simulink model "Switchvideo_orientation"  (R2024a)
settings: Solver=FixedStepAuto  StartTime=0.0  StopTime=inf  RelTol=1e-3
undefined symbols (not defined in the file): VideoDirection
settings Model: Creator=Sasha  LastModifiedBy=quentinlandon

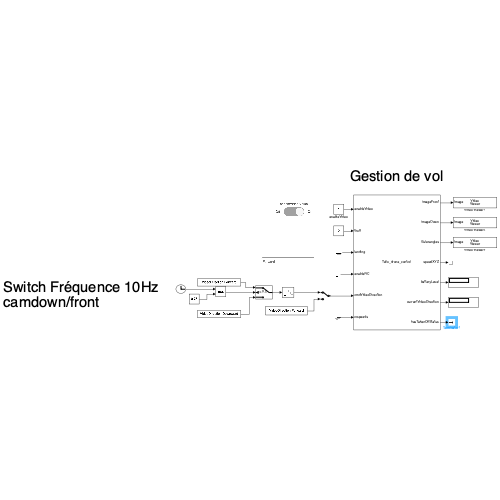
[thumbnail: Simulink's stored preview of the top-level diagram]
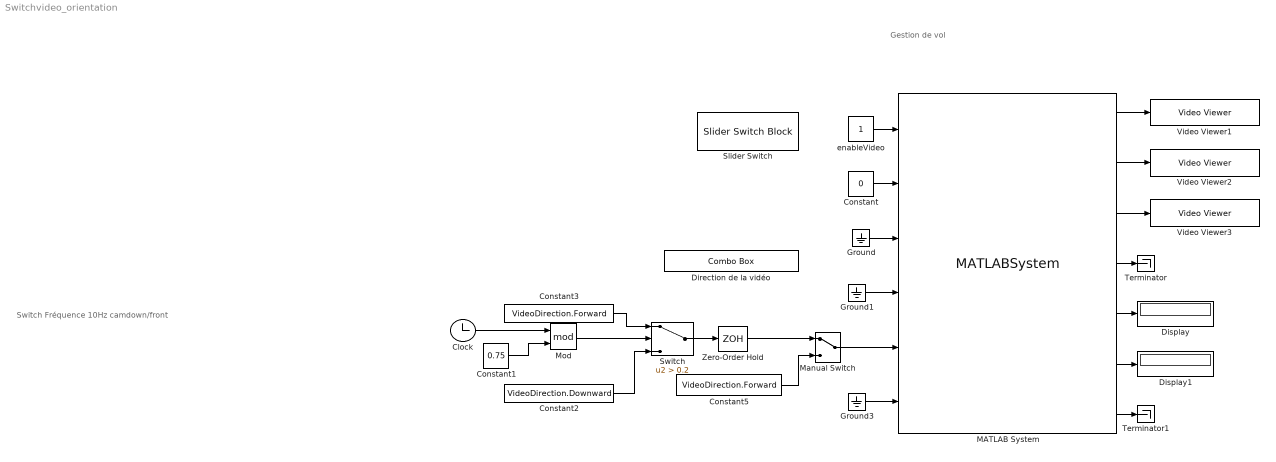
== system Switchvideo_orientation ==
  note: Gestion de vol
  note: Switch Fréquence 10Hz camdown/front
  Clock : Clock
  Constant : Constant  Value=0
  Constant1 : Constant  Value=0.75
  Constant2 : Constant  Value=VideoDirection.Downward
  Constant3 : Constant  Value=VideoDirection.Forward
  Constant5 : Constant  Value=VideoDirection.Forward
  Direction de la vidéo : ComboBox  LabelPosition=Hide  SelectedLabel=Forward  UseEnumeratedDataType=on  EnumeratedDataType=VideoDirection
      settings: Values={{'Forward', 'Downward', 'Both'}, [0 1 2]}
  Display : Display
  Display1 : Display
  Ground : Ground
  Ground1 : Ground
  Ground3 : Ground
  MATLAB System : MATLABSystem  System=Tello_drone_control  droneIP=127.0.0.1  SimulateUsing=Interpreted execution
      mask Type: Tello_drone_control
      mask Display:
      | disp('Tello_drone_control');
      | port_label('input',1,'enableVideo');
      | port_label('input',2,'tkoff');
      | port_label('input',3,'landing');
      | port_label('input',4,'enableRC');
      | port_label('input',5,'cmdVideoDirection');
      | port_label('input',6,'rcspeeds');
      | port_label('output',1,'imageFront');
      | port_label('output',2,'imageDown');
      | port_label('output',3,'Eulerangles');
      | port_label('output',4,'speedXYZ');
      | port_label('output',5,'batteryLevel');
      | port_label('output',6,'currentVideoDirection');
      | port_label('output',7,'hasTakenOffStatus');
  Manual Switch : ManualSwitch
  Mod : Math  Operator=mod
  Slider Switch : SliderSwitchBlock
      settings: Values={{'Off', 'On'}, [0 1]}
  Switch : Switch  Criteria=u2 > Threshold  Threshold=0.2  SaturateOnIntegerOverflow=off  InputSameDT=off
  Terminator : Terminator
  Terminator1 : Terminator
  Video Viewer1 : VideoViewer  FigPos=[691 499 750 371]
  Video Viewer2 : VideoViewer  FigPos=[691 836 750 371]
  Video Viewer3 : VideoViewer  FigPos=[128.333333333333 836 1080.66666666667 580]
  Zero-Order Hold : ZeroOrderHold  SampleTime=-1
  enableVideo : Constant
  wires:
  enableVideo/1 -> MATLAB System/1
  MATLAB System/1 -> Video Viewer1/1
  MATLAB System/2 -> Video Viewer2/1
  MATLAB System/3 -> Video Viewer3/1
  Constant/1 -> MATLAB System/2
  Constant1/1 -> Mod/2
  Mod/1 -> Switch/2
  Constant2/1 -> Switch/3
  Constant3/1 -> Switch/1
  Switch/1 -> Zero-Order Hold/1
  Zero-Order Hold/1 -> Manual Switch/1
  Clock/1 -> Mod/1
  Manual Switch/1 -> MATLAB System/5
  Constant5/1 -> Manual Switch/2
  MATLAB System/5 -> Display/1
  MATLAB System/4 -> Terminator/1
  MATLAB System/6 -> Display1/1
  MATLAB System/7 -> Terminator1/1
  Ground/1 -> MATLAB System/3
  Ground1/1 -> MATLAB System/4
  Ground3/1 -> MATLAB System/6
